simulink model "model_linear_mpc"  (R2022a)
settings: Solver=VariableStepAuto  StartTime=0  StopTime=100  RelTol=1e-3
values from neighbouring files (symbols this model uses):
  A = [ 0 1 0  0 ... (first row only)    [ball_and_beam_pfc.m]
  amplitude_entrada = 1    [ball_and_beam_pfc.m]
  B = [0 ... (first row only)    [ball_and_beam_pfc.m]
  bool_degrau = 1    [ball_and_beam_pfc.m]
  C = [0 0 1 0]    [ball_and_beam_pfc.m]
  L = 0.425    [ball_and_beam_pfc.m]    (also in nonlinear_ball_and_beam.m)
libraries: vrlib x3, mpclib x1
settings Model: Creator=Notebook_Artur  LastModifiedBy=Notebook_Artur

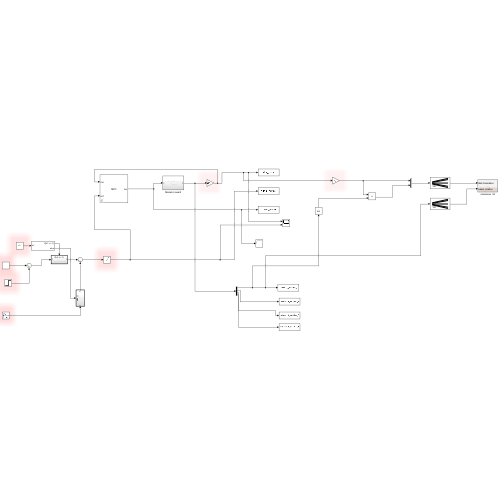
[thumbnail: Simulink's stored preview of the top-level diagram]
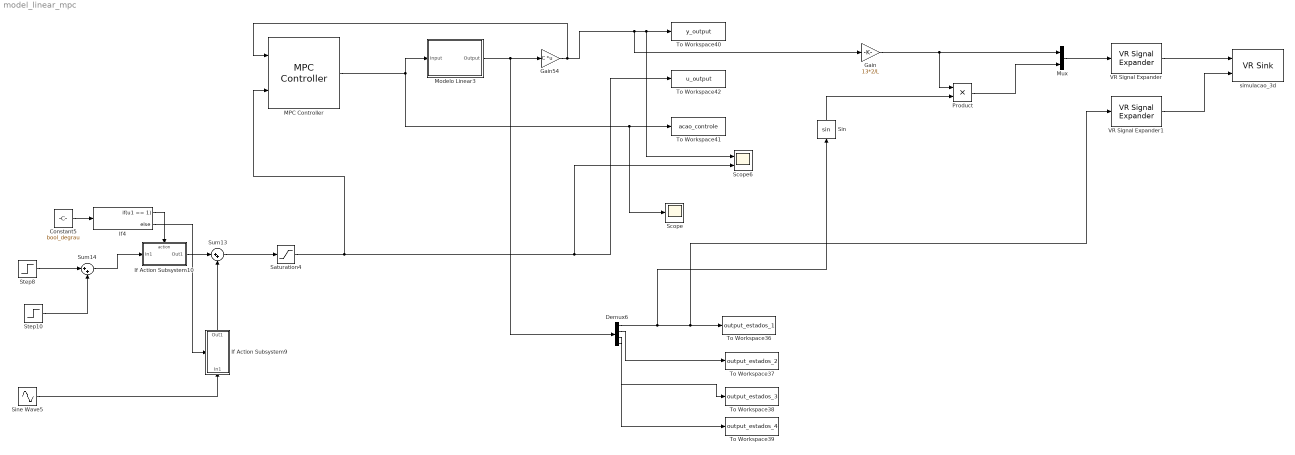
== system model_linear_mpc ==
  Constant5 : Constant  Value=bool_degrau
  Demux6 : Demux
  Gain : Gain  Gain=13*2/L
  Gain54 : Gain  Gain=C  Multiplication=Matrix(K*u)
  If Action Subsystem10 : Subsystem  TreatAsAtomicUnit=on
  If Action Subsystem9 : Subsystem  TreatAsAtomicUnit=on
  If4 : If  IfExpression=u1 == 1
  MPC Controller : mpclib/MPC Controller  SCDEnableBlockLinearizationSpecification=on  mpcobj=mpc1  is_multiple=0  enable_value=0  return_u0=off  updateMPCinCallerWorkspace=on  md_inport=off  mv_inport=off  uref_inport=off  return_cost=off  return_mvseq=off  return_qpstatus=off  return_xseq=off  return_state=off  return_ovseq=off  state_inport=off  umin_inport=off  umax_inport=off  ymin_inport=off  ymax_inport=off  cc_inport=off  ywt_inport=off  uwt_inport=off  duwt_inport=off  rhoeps_inport=off  pm_inport=off  MaximumP=10  HorizonChoice=FixedHorizon  n_ts=0.1  n_p=10  n_mv=1  n_md=0  n_ud=0  n_mo=1  n_uo=0  BlockDataType=double  SampleTimeInherited=off  switch_inport=off
  Modelo Linear3 : Subsystem
  Mux : Mux  Inputs=2
  Product : Product
  Saturation4 : Saturate  UpperLimit=L/2  LowerLimit=-L/2
  Scope : Scope
  Scope6 : Scope  NumInputPorts=2
  Sin : Trigonometry
  Sine Wave5 : Sin  Amplitude=amplitude_entrada  Frequency=0.1  SampleTime=0
  Step10 : Step  Time=100  After=-2*amplitude_entrada  SampleTime=0
  Step8 : Step  After=amplitude_entrada  SampleTime=0
  Sum13 : Sum  Inputs=|++
  Sum14 : Sum  Inputs=|++
  To Workspace36 : ToWorkspace  VariableName=output_estados_1  SaveFormat=Timeseries  SampleTime=-1
  To Workspace37 : ToWorkspace  VariableName=output_estados_2  SaveFormat=Timeseries  SampleTime=-1
  To Workspace38 : ToWorkspace  VariableName=output_estados_3  SaveFormat=Timeseries  SampleTime=-1
  To Workspace39 : ToWorkspace  VariableName=output_estados_4  SaveFormat=Timeseries  SampleTime=-1
  To Workspace40 : ToWorkspace  VariableName=y_output  SaveFormat=Timeseries  SampleTime=-1
  To Workspace41 : ToWorkspace  VariableName=acao_controle  SaveFormat=Timeseries  SampleTime=-1
  To Workspace42 : ToWorkspace  VariableName=u_output  SaveFormat=Timeseries  SampleTime=-1
  VR Signal Expander : vrlib/VR Signal Expander  outwidth=3  outidx=[1 3]
  VR Signal Expander1 : vrlib/VR Signal Expander  outwidth=4  outidx=[4]
  simulacao_3d : vrlib/VR Sink  InstantiateOnLoad=on  SampleTime=0.1  ViewEnable=on  RemoteChange=off  RemoteView=off  FieldsWritten=Ball.translation.3.1.1.double#beam.rotation.4.1.1.double  WorldFileName=3d_ball_and_beam4.x3d  AutoView=on  VideoDimensions=[]  AllowVariableSize=off
  wires:
  MPC Controller/1 -> Scope/1, To Workspace41/1, Modelo Linear3/1(Input)
  Saturation4/1 -> MPC Controller/2, Scope6/2, To Workspace42/1
  Step10/1 -> Sum14/2
  If4/2 -> If Action Subsystem9/Action
  If Action Subsystem9/1(Out1) -> Sum13/2
  Modelo Linear3/1(Output) -> Demux6/1, Gain54/1
  If4/1 -> If Action Subsystem10/Action
  Sine Wave5/1 -> If Action Subsystem9/1(In1)
  Demux6/3 -> To Workspace38/1
  Demux6/4 -> To Workspace39/1
  Sum13/1 -> Saturation4/1
  If Action Subsystem10/1(Out1) -> Sum13/1
  Demux6/2 -> To Workspace37/1
  Sum14/1 -> If Action Subsystem10/1(In1)
  Step8/1 -> Sum14/1
  Constant5/1 -> If4/1
  Demux6/1 -> VR Signal Expander1/1, To Workspace36/1, Sin/1
  VR Signal Expander/1 -> simulacao_3d/1
  VR Signal Expander1/1 -> simulacao_3d/2
  Product/1 -> Mux/2
  Gain/1 -> Mux/1, Product/1
  Mux/1 -> VR Signal Expander/1
  Sin/1 -> Product/2
  Gain54/1 -> MPC Controller/1, Gain/1, Scope6/1, To Workspace40/1

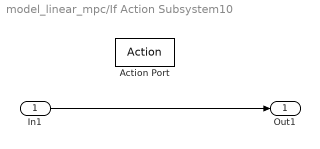
== system model_linear_mpc/If Action Subsystem10 ==
  In1 : Inport
  Action Port : ActionPort  ActionPortLabel=if(u1 == 1)
  Out1 : Outport
  wires:
  In1/1 -> Out1/1

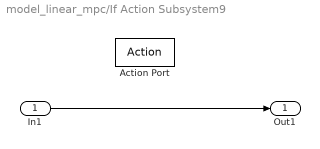
== system model_linear_mpc/If Action Subsystem9 ==
  In1 : Inport
  Action Port : ActionPort  ActionPortLabel=else
  Out1 : Outport
  wires:
  In1/1 -> Out1/1

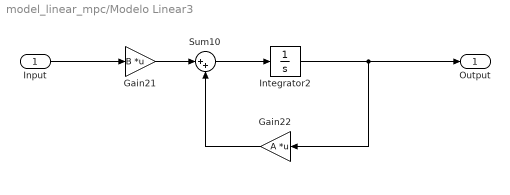
== system model_linear_mpc/Modelo Linear3 ==
  Input : Inport
  Gain21 : Gain  Gain=B  Multiplication=Matrix(K*u)
  Gain22 : Gain  Gain=A  Multiplication=Matrix(K*u)
  Integrator2 : Integrator
  Sum10 : Sum  Inputs=|++
  Output : Outport
  wires:
  Input/1 -> Gain21/1
  Gain22/1 -> Sum10/2
  Integrator2/1 -> Output/1, Gain22/1
  Gain21/1 -> Sum10/1
  Sum10/1 -> Integrator2/1
